simulink model "combinedTxRx"  (R2017b)
settings: Solver=FixedStepDiscrete  StartTime=0.0  StopTime=10.0  RelTol=1e-3
InitFcn:
  | modelSettings
undefined symbols (not defined in the file or in its folder): RadioSampleRate
libraries: RxTxFixedPointLibrary x2, dspsigops x2, commsource2 x1
settings Model: Creator=tcollins  LastModifiedBy=tcollins
settings OptimizationCC: BlockReduction=off  ConditionallyExecuteInputs=off  DefaultParameterBehavior=Inlined
settings DebuggingCC: AlgebraicLoopMsg=error  SingleTaskRateTransMsg=error  ParameterPrecisionLossMsg=none
settings HardwareCC: ProdBitPerPointer=32  ProdBitPerSizeT=32  ProdBitPerPtrDiffT=32  ProdLargestAtomicFloat=None  ProdIntDivRoundTo=Undefined  ProdEndianess=Unspecified  ProdWordSize=32  ProdHWDeviceType=ASIC/FPGA->ASIC/FPGA  ProdEqTarget=off
settings CodeAppCC: StateflowObjectComments=on

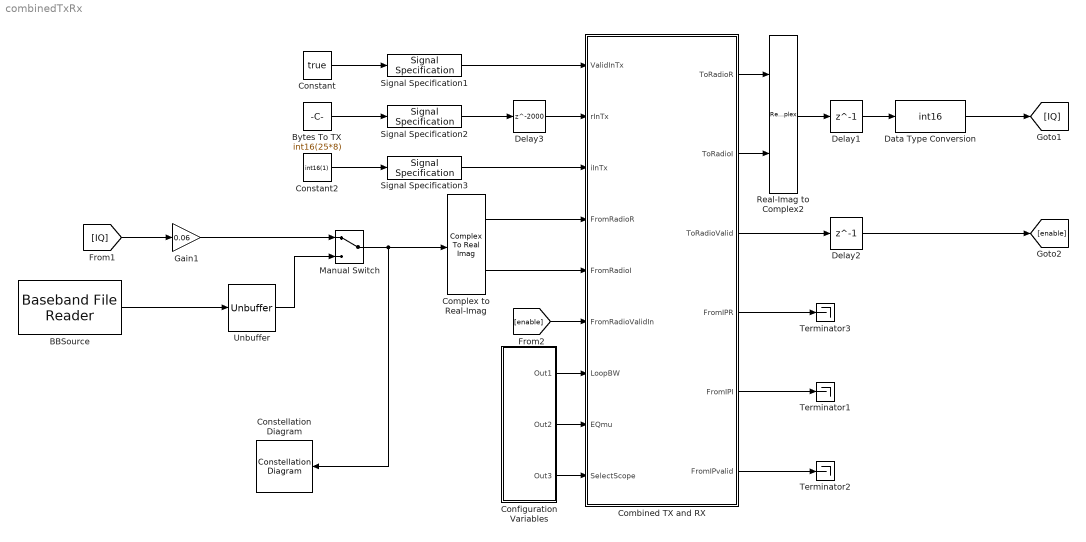
== system combinedTxRx ==
  BBSource : commsource2/Baseband File Reader  Filename=PlutoCaptureQPSK.bb  InheritSampleTimeFromFile=off  SampleTime=100000/(RadioSampleRate)  SamplesPerFrame=100000  CyclicRepetition=off  FileEndOutputPort=off  SimulateUsing=Interpreted execution
      settings: SourceProductName=Communications System Toolbox  SourceProductBaseCode=CM
  Bytes To TX : Constant  Value=int16(25*8)  SampleTime=-1
  Combined TX and RX : Subsystem  TreatAsAtomicUnit=on
  Complex to Real-Imag : ComplexToRealImag
  Configuration Variables : Subsystem
  Constant : Constant  Value=true  SampleTime=-1
  Constant2 : Constant  Value=int16(1)  SampleTime=-1
  Constellation Diagram : ConstellationDiagram
  Data Type Conversion : DataTypeConversion  OutDataTypeStr=int16  ConvertRealWorld=Stored Integer (SI)
  Delay1 : Delay  DelayLength=1
  Delay2 : Delay  DelayLength=1
  Delay3 : Delay  DelayLength=2000
  Gain1 : Gain  Gain=0.06  OutDataTypeStr=int16
  Manual Switch : ManualSwitch
  Real-Imag to Complex2 : RealImagToComplex
  Signal Specification1 : SignalSpecification  OutDataTypeStr=boolean  SampleTime=1/RadioSampleRate
  Signal Specification2 : SignalSpecification  OutDataTypeStr=int16  SampleTime=1/RadioSampleRate
  Signal Specification3 : SignalSpecification  OutDataTypeStr=int16  SampleTime=1/RadioSampleRate
  Terminator1 : Terminator
  Terminator2 : Terminator
  Terminator3 : Terminator
  Unbuffer : Unbuffer
  wires:
  Bytes To TX/1 -> Signal Specification2/1
  Constant2/1 -> Signal Specification3/1
  Constant/1 -> Signal Specification1/1
  BBSource/1 -> Unbuffer/1
  Signal Specification1/1 -> Combined TX and RX/1(ValidInTx)
  Signal Specification2/1 -> Delay3/1
  Signal Specification3/1 -> Combined TX and RX/3(iInTx)
  [enable] -> Combined TX and RX/6(FromRadioValidIn)
  Combined TX and RX/3(ToRadioValid) -> Delay2/1
  Delay1/1 -> Data Type Conversion/1
  Data Type Conversion/1 -> [IQ]
  Delay2/1 -> [enable]
  Manual Switch/1 -> Constellation Diagram/1, Complex to Real-Imag/1
  Delay3/1 -> Combined TX and RX/2(rInTx)
  [IQ] -> Gain1/1
  Gain1/1 -> Manual Switch/1
  Complex to Real-Imag/1 -> Combined TX and RX/4(FromRadioR)
  Complex to Real-Imag/2 -> Combined TX and RX/5(FromRadioI)
  Unbuffer/1 -> Manual Switch/2
  Combined TX and RX/1(ToRadioR) -> Real-Imag to Complex2/1
  Combined TX and RX/2(ToRadioI) -> Real-Imag to Complex2/2
  Real-Imag to Complex2/1 -> Delay1/1
  Configuration Variables/1(Out1) -> Combined TX and RX/7(LoopBW)
  Configuration Variables/2(Out2) -> Combined TX and RX/8(EQmu)
  Configuration Variables/3(Out3) -> Combined TX and RX/9(SelectScope)
  Combined TX and RX/4(FromIPR) -> Terminator3/1
  Combined TX and RX/5(FromIPI) -> Terminator1/1
  Combined TX and RX/6(FromIPvalid) -> Terminator2/1

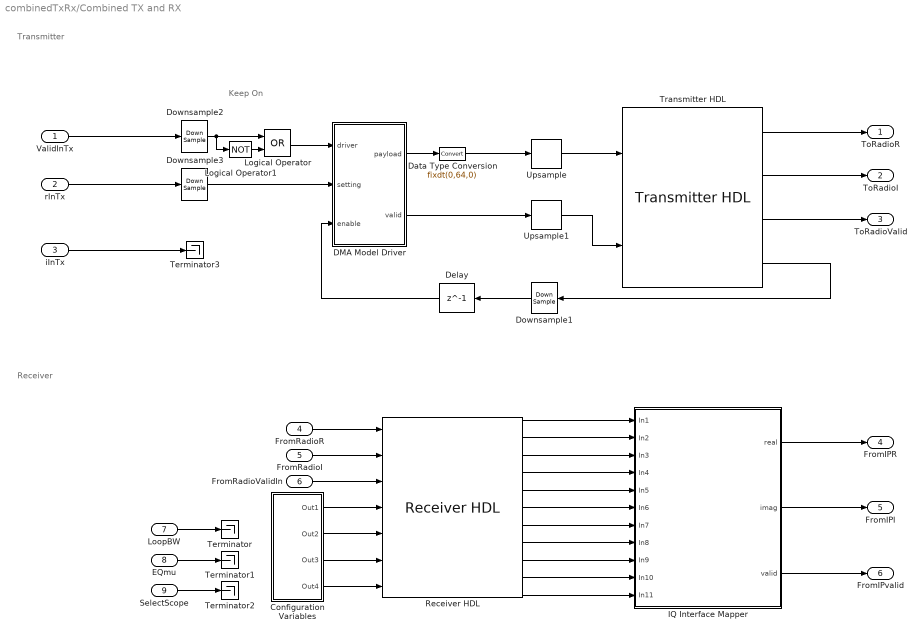
== system combinedTxRx/Combined TX and RX ==
  note: Receiver
  note: Transmitter
  note: Keep On
  ValidInTx : Inport
  rInTx : Inport  Port=2
  iInTx : Inport  Port=3
  FromRadioR : Inport  Port=4  PortDimensions=1
  FromRadioI : Inport  Port=5  PortDimensions=1
  FromRadioValidIn : Inport  Port=6
  LoopBW : Inport  Port=7
  EQmu : Inport  Port=8
  SelectScope : Inport  Port=9
  Configuration Variables : Subsystem
  DMA Model Driver : MATLAB Function  TreatAsAtomicUnit=on
  Data Type Conversion : DataTypeConversion  OutDataTypeStr=fixdt(0,64,0)
  Delay : Delay  DelayLength=1
  Downsample1 : DownSample  N=4  RateOptions=Allow multirate processing
  Downsample2 : DownSample  N=4  RateOptions=Allow multirate processing
  Downsample3 : DownSample  N=4  RateOptions=Allow multirate processing
  IQ Interface Mapper : Subsystem
  Logical Operator : Logic  Operator=OR  AllPortsSameDT=off  OutDataTypeStr=boolean
  Logical Operator1 : Logic  Operator=NOT  AllPortsSameDT=off  OutDataTypeStr=boolean
  Receiver HDL : RxTxFixedPointLibrary/Receiver HDL  SystemSampleTime=-1
  Terminator{,1..3} (4 alike) : Terminator
  Transmitter HDL : RxTxFixedPointLibrary/Transmitter HDL  SystemSampleTime=-1
  Upsample : dspsigops/Upsample  N=4  phase=0  RateOptions=Allow multirate processing  ic=0  mode=Unused parameter value
  Upsample1 : dspsigops/Upsample  N=4  phase=0  RateOptions=Allow multirate processing  ic=0  mode=Unused parameter value
  ToRadioR : Outport
  ToRadioI : Outport  Port=2
  ToRadioValid : Outport  Port=3
  FromIPR : Outport  Port=4
  FromIPI : Outport  Port=5
  FromIPvalid : Outport  Port=6
  wires:
  FromRadioValidIn/1 -> Receiver HDL/3
  FromRadioR/1 -> Receiver HDL/1
  rInTx/1 -> Downsample3/1
  Transmitter HDL/2 -> ToRadioI/1
  Transmitter HDL/3 -> ToRadioValid/1
  Transmitter HDL/1 -> ToRadioR/1
  iInTx/1 -> Terminator3/1
  ValidInTx/1 -> Downsample2/1
  FromRadioI/1 -> Receiver HDL/2
  LoopBW/1 -> Terminator/1
  EQmu/1 -> Terminator1/1
  SelectScope/1 -> Terminator2/1
  Configuration Variables/1(Out1) -> Receiver HDL/4
  Configuration Variables/2(Out2) -> Receiver HDL/5
  Configuration Variables/3(Out3) -> Receiver HDL/6
  Downsample3/1 -> DMA Model Driver/2(setting)
  Data Type Conversion/1 -> Upsample/1
  Delay/1 -> DMA Model Driver/3(enable)
  DMA Model Driver/1(payload) -> Data Type Conversion/1
  Downsample1/1 -> Delay/1
  DMA Model Driver/2(valid) -> Upsample1/1
  Downsample2/1 -> Logical Operator/1, Logical Operator1/1
  Logical Operator/1 -> DMA Model Driver/1(driver)
  Logical Operator1/1 -> Logical Operator/2
  Transmitter HDL/4 -> Downsample1/1
  Upsample1/1 -> Transmitter HDL/2
  Upsample/1 -> Transmitter HDL/1
  Receiver HDL/1 -> IQ Interface Mapper/1(In1)
  Receiver HDL/2 -> IQ Interface Mapper/2(In2)
  Receiver HDL/3 -> IQ Interface Mapper/3(In3)
  Receiver HDL/4 -> IQ Interface Mapper/4(In4)
  Receiver HDL/5 -> IQ Interface Mapper/5(In5)
  Receiver HDL/6 -> IQ Interface Mapper/6(In6)
  Receiver HDL/7 -> IQ Interface Mapper/7(In7)
  Receiver HDL/8 -> IQ Interface Mapper/8(In8)
  Receiver HDL/9 -> IQ Interface Mapper/9(In9)
  IQ Interface Mapper/1(real) -> FromIPR/1
  IQ Interface Mapper/2(imag) -> FromIPI/1
  IQ Interface Mapper/3(valid) -> FromIPvalid/1
  Receiver HDL/10 -> IQ Interface Mapper/10(In10)
  Configuration Variables/4(Out4) -> Receiver HDL/7
  Receiver HDL/11 -> IQ Interface Mapper/11(In11)

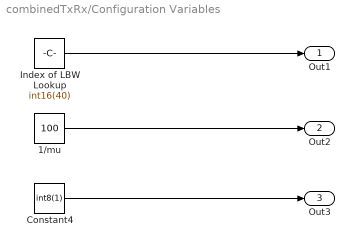
== system combinedTxRx/Configuration Variables ==
  1/mu : Constant  Value=100  OutDataTypeStr=int16  SampleTime=-1
  Constant4 : Constant  Value=int8(1)  SampleTime=1/RadioSampleRate
  Index of LBW Lookup : Constant  Value=int16(40)  SampleTime=1/RadioSampleRate
  Out1 : Outport
  Out2 : Outport  Port=2
  Out3 : Outport  Port=3
  wires:
  1/mu/1 -> Out2/1
  Index of LBW Lookup/1 -> Out1/1
  Constant4/1 -> Out3/1

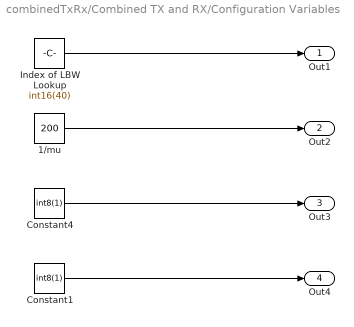
== system combinedTxRx/Combined TX and RX/Configuration Variables ==
  1/mu : Constant  Value=200  OutDataTypeStr=int16  SampleTime=-1
  Constant1 : Constant  Value=int8(1)  SampleTime=1/RadioSampleRate
  Constant4 : Constant  Value=int8(1)  SampleTime=1/RadioSampleRate
  Index of LBW Lookup : Constant  Value=int16(40)  SampleTime=1/RadioSampleRate
  Out1 : Outport
  Out2 : Outport  Port=2
  Out3 : Outport  Port=3
  Out4 : Outport  Port=4
  wires:
  1/mu/1 -> Out2/1
  Index of LBW Lookup/1 -> Out1/1
  Constant4/1 -> Out3/1
  Constant1/1 -> Out4/1

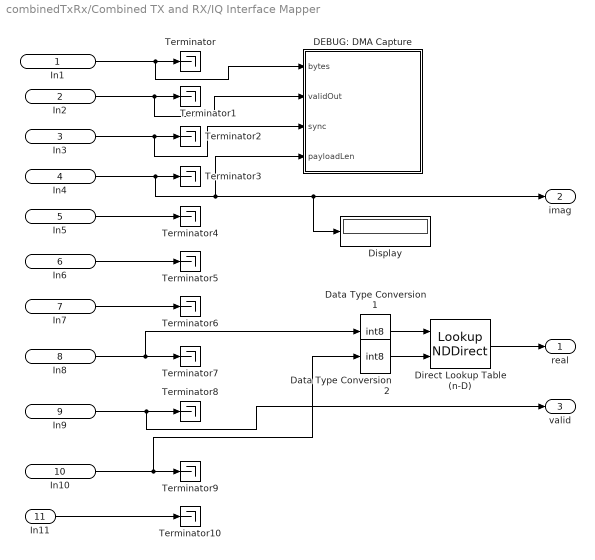
== system combinedTxRx/Combined TX and RX/IQ Interface Mapper ==
  In1 : Inport
  In2 : Inport  Port=2
  In3 : Inport  Port=3
  In4 : Inport  Port=4
  In5 : Inport  Port=5
  In6 : Inport  Port=6
  In7 : Inport  Port=7
  In8 : Inport  Port=8
  In9 : Inport  Port=9
  In10 : Inport  Port=10
  In11 : Inport  Port=11
  DEBUG: DMA Capture : MATLAB Function  TreatAsAtomicUnit=on
  Data Type Conversion1 : DataTypeConversion  OutDataTypeStr=int8
  Data Type Conversion2 : DataTypeConversion  OutDataTypeStr=int8
  Direct Lookup Table (n-D) : LookupNDDirect  Table=[1 2; 3 4]  DiagnosticForOutOfRangeInput=Error  TableDataTypeStr=int16
  Display : Display
  Terminator{,1..10} (11 alike) : Terminator
  real : Outport
  imag : Outport  Port=2
  valid : Outport  Port=3
  wires:
  Data Type Conversion1/1 -> Direct Lookup Table (n-D)/1
  Data Type Conversion2/1 -> Direct Lookup Table (n-D)/2
  Direct Lookup Table (n-D)/1 -> real/1
  In1/1 -> DEBUG: DMA Capture/1(bytes), Terminator/1
  In2/1 -> DEBUG: DMA Capture/2(validOut), Terminator1/1
  In3/1 -> DEBUG: DMA Capture/3(sync), Terminator2/1
  In4/1 -> DEBUG: DMA Capture/4(payloadLen), Display/1, imag/1, Terminator3/1
  In5/1 -> Terminator4/1
  In6/1 -> Terminator5/1
  In7/1 -> Terminator6/1
  In8/1 -> Data Type Conversion1/1, Terminator7/1
  In9/1 -> valid/1, Terminator8/1
  In10/1 -> Data Type Conversion2/1, Terminator9/1
  In11/1 -> Terminator10/1

== matlab function combinedTxRx/Combined TX and RX/IQ Interface Mapper/DEBUG: DMA Capture ==
  data: bytes input; validOut input; sync input; payloadLen input
function fcn(bytes, validOut, sync, payloadLen)

persistent frameBuffer byteCounter fullPayloadBits

bitsInPack = 64;

if isempty(frameBuffer)
    maxFrameBits = (2^16)*8;
    frameBuffer = false(maxFrameBits,1);
    byteCounter = 0;
    fullPayloadBits = uint16(0);
end

if validOut
    if sync
        byteCounter = bitsInPack;
        frameBuffer(1:byteCounter) = bitget(bytes,1:bitsInPack);
        fullPayloadBits = uint16(payloadLen*8);
        
    elseif byteCounter<fullPayloadBits
        frameBuffer(byteCounter+1:byteCounter+bitsInPack) = bitget(bytes,1:bitsInPack);
        byteCounter = byteCounter + bitsInPack;
    else
        if bytes>0
            disp('CRC Error (Outside)');
        else
            disp('Frame passed CRC (Outside)');
        end
    end
end

== matlab function combinedTxRx/Combined TX and RX/DMA Model Driver ==
  data: driver input; setting input; payload output; valid output boolean; enable input
function [payload,valid] = fcn(driver, setting, enable)
%#codegen

persistent indx mode pSize

if isempty(indx)
    pSize = fi(200,0,64,0); % Size in bytes (Must be multiple of 32 bits) cannot exceed uint16 max
    indx = pSize;
    mode = int8(0);
end


if enable && driver
    valid = true;
    switch mode
        case int8(0) % Fresh packet start
            if setting>0
                pSize = fi(setting,0,64,0);
                payload = fi(setting,0,64,0);%Upper bits
                mode = int8(1);
                indx = fi(0,0,64,0);
                %fprintf('(TX) Sending new packet with length: %u\n',uint64(pSize));
            else
                valid = false;
                payload = fi(0,0,64,0);
            end
        otherwise
            indx = fi(indx + fi(8,0,64,0),0,64,0);
            if indx == fi(8,0,64,0)
               payload = fi(0,0,64,0);
               payload = bitset(payload,1,1);
%                 payload = fi(uint64(12297829382473034410),0,64,0);%sum(2.^[0:2:14])); % Alternating ones and zeros
            elseif indx == pSize
                payload = fi(uint64(18446744073709551615),0,64,0); % All ones
%                  payload = fi(uint64(12297829382473034410),0,64,0);%sum(2.^[0:2:14])); % Alternating ones and zeros
          else
                %payload = fi(uint64(randi([0 12297829382473034410])),0,64,0);%sum(2.^[0:2:14])); % Alternating ones and zeros
                payload = fi(uint64(12297829382473034410),0,64,0);%sum(2.^[0:2:14])); % Alternating ones and zeros
            end
            if indx == pSize % reached end of frame
                mode = int8(0);
            end
    end
else
    valid = false;
    payload = fi(0,0,64,0);
end
